simulink model "Meas_Noise_Test"  (R2022a)
settings: Solver=FixedStepAuto  StartTime=tspan(1)  StopTime=tspan(2)  FixedStep=Ts  RelTol=1e-9
undefined symbols (not defined in the file): Serial_Port, Standard_Devices, Ts
libraries: simulink_extras x4, sldrtlib x2, simulink x1, cstblocks x1
settings Model: SimulationMode=external  Creator=zachn  LastModifiedBy=domin
settings SolverCC: AlgebraicLoopSolver=TrustRegion
settings DataIOCC: SaveFormat=StructureWithTime  InspectSignalLogs=on
settings DebuggingCC: UnconnectedInputMsg=warning  UnconnectedOutputMsg=warning  UnconnectedLineMsg=warning  SFMachineParentedDataDiag=warning
settings HardwareCC: ProdBitPerLong=64  ProdHWDeviceType=Intel->x86-64 (Linux 64)
settings RTWCC: Description=Simulink Desktop Real-Time  SystemTargetFile=sldrt.tlc  TemplateMakefile=sldrt.tmf  RTWCompilerOptimization=on  DLArmComputeVersion=19.05
settings CodeAppCC: MaxIdLength=95
settings SimulinkDesktopRealTimeCC: TargetLibSuffix=_sldrt.a  TargetPreCompLibLocation=C:\Program Files\MATLAB\R2022a\toolbox\sldrt\lib\win64

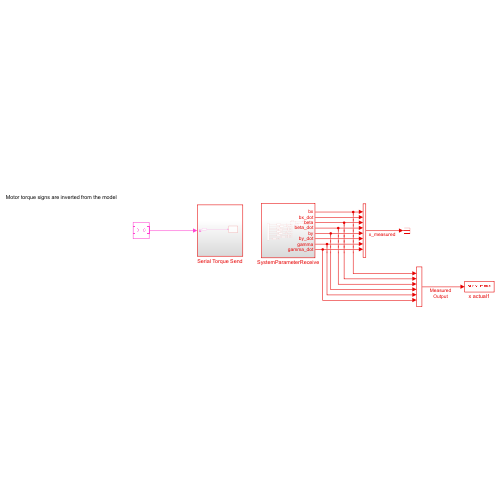
[thumbnail: Simulink's stored preview of the top-level diagram]
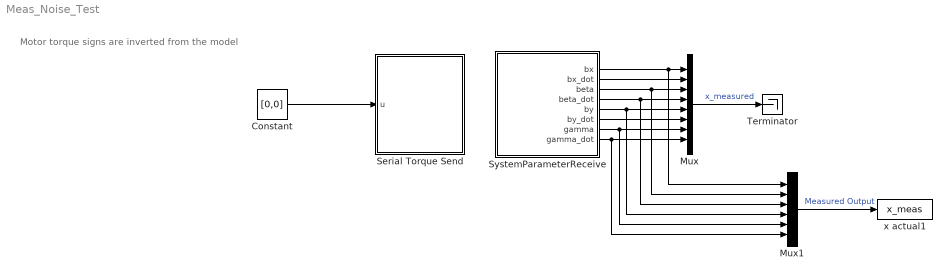
== system Meas_Noise_Test ==
  note: Motor torque signs are inverted from the model
  Constant : Constant  Value=[0,0]
  Mux : Mux  Inputs=8
  Mux1 : Mux  Inputs=6
  Serial Torque Send : Subsystem
  SystemParameterReceive : Subsystem
  Terminator : Terminator
  x actual1 : ToWorkspace  VariableName=x_meas  SampleTime=Ts
  wires:
  Constant/1 -> Serial Torque Send/1(u)
  SystemParameterReceive/6(by_dot) -> Mux/6
  SystemParameterReceive/2(bx_dot) -> Mux/2
  SystemParameterReceive/3(beta) -> Mux1/2, Mux/3
  SystemParameterReceive/5(by) -> Mux1/4, Mux/5
  Mux1/1 -> x actual1/1  "Measured Output"
  SystemParameterReceive/1(bx) -> Mux1/1, Mux/1
  SystemParameterReceive/8(gamma_dot) -> Mux1/6, Mux/8
  SystemParameterReceive/7(gamma) -> Mux1/5, Mux/7
  SystemParameterReceive/4(beta_dot) -> Mux1/3, Mux/4
  Mux/1 -> Terminator/1  "x_measured"

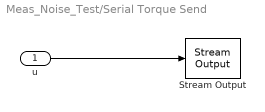
== system Meas_Noise_Test/Serial Torque Send ==
  u : Inport
  Stream Output : sldrtlib/Stream Output  SampleTime=Ts  MaxMissedTicks=10  ShowMissedTicks=off  YieldWhenWaiting=off  DrvName=Standard_Devices/Serial_Port  DrvAddress=6  DrvOptions=[115200 8 0 0 1 0 0 0]  PortSizes=2  FormatString='%g %g\n'  ShowReady=off  ShowError=off  InitialValue=[]  FinalValue=[]
      settings: AttributesFormatString=Serial Port [6]  SourceProductBaseCode=WT
  wires:
  u/1 -> Stream Output/1

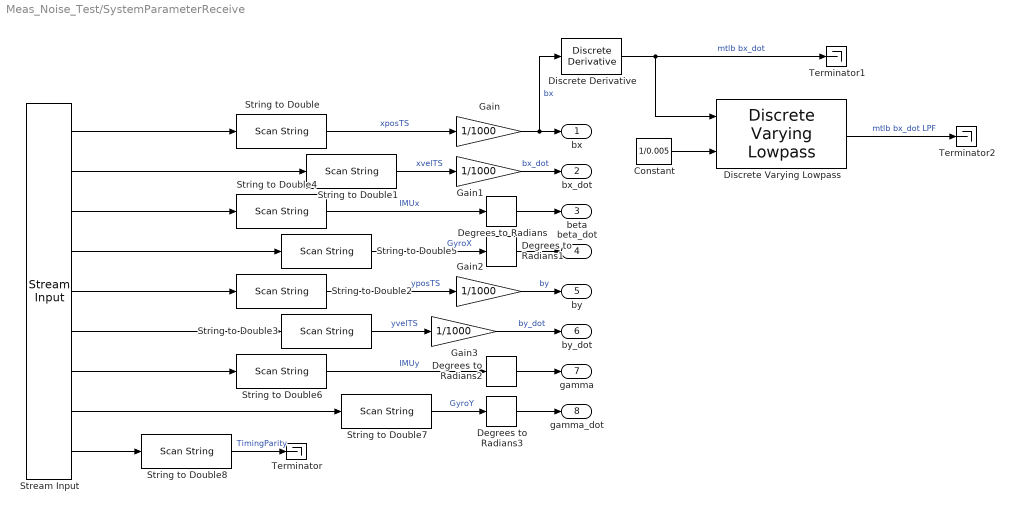
== system Meas_Noise_Test/SystemParameterReceive ==
  Constant : Constant  Value=1/0.005
  Degrees to Radians{,1..3} (4 alike) : simulink_extras/Transformations/Degrees to Radians
  Discrete Derivative : simulink/Discrete/Discrete Derivative  gainval=1.0  ICPrevScaledInput=0.0  OutMin=[]  OutMax=[]  OutDataType=fixdt(1, 16)  OutScaling=2^-10  DoSatur=off
  Discrete Varying Lowpass : cstblocks/Linear Parameter Varying/Discrete Varying Lowpass  N=4  w0=0  Ts=Ts
      settings: SourceProductBaseCode=CT
  Gain{,1..3} (4 alike) : Gain  Gain=1/1000  OutDataTypeStr=double
  Stream Input : sldrtlib/Stream Input  SampleTime=Ts  MaxMissedTicks=10  ShowMissedTicks=off  YieldWhenWaiting=on  DrvName=Standard_Devices/Serial_Port  DrvAddress=6  DrvOptions=[115200 8 0 0 1 0 0 0]  DataTypes={'string','string','string','string','string','string','string','string','string'}  FormatString='%s %s %s %s %s %s %s %s %s'  Terminator={'\r', '\n'}  ShowReady=off  ShowError=off
      settings: AttributesFormatString=Serial Port [6]  SourceProductBaseCode=WT
  String to Double : ScanString  Format="\"%d\""
  String to Double{1..8} (8 alike) : ScanString  Format="\"%lf\""
  Terminator : Terminator
  Terminator1 : Terminator
  Terminator2 : Terminator
  bx : Outport
  bx_dot : Outport  Port=2
  beta : Outport  Port=3
  beta_dot : Outport  Port=4
  by : Outport  Port=5
  by_dot : Outport  Port=6
  gamma : Outport  Port=7
  gamma_dot : Outport  Port=8
  wires:
  Stream Input/1 -> String to Double/1
  Stream Input/8 -> String to Double7/1
  Degrees to Radians3/1 -> gamma_dot/1
  Degrees to Radians2/1 -> gamma/1
  Stream Input/6 -> String to Double3/1
  Stream Input/9 -> String to Double8/1
  Stream Input/5 -> String to Double2/1
  String to Double8/1 -> Terminator/1  "TimingParity"
  Stream Input/7 -> String to Double6/1
  String to Double6/1 -> Degrees to Radians2/1  "IMUy"
  Stream Input/2 -> String to Double1/1
  String to Double1/1 -> Gain1/1  "xvelTS"
  Gain1/1 -> bx_dot/1  "bx_dot"
  Stream Input/4 -> String to Double5/1
  Stream Input/3 -> String to Double4/1
  Gain/1 -> Discrete Derivative/1, bx/1  "bx"
  String to Double/1 -> Gain/1  "xposTS"
  String to Double7/1 -> Degrees to Radians3/1  "GyroY"
  String to Double2/1 -> Gain2/1  "yposTS"
  Gain2/1 -> by/1  "by"
  Gain3/1 -> by_dot/1  "by_dot"
  String to Double3/1 -> Gain3/1  "yvelTS"
  Degrees to Radians1/1 -> beta_dot/1
  Degrees to Radians/1 -> beta/1
  String to Double4/1 -> Degrees to Radians/1  "IMUx"
  String to Double5/1 -> Degrees to Radians1/1  "GyroX"
  Discrete Derivative/1 -> Discrete Varying Lowpass/1, Terminator1/1  "mtlb bx_dot"
  Constant/1 -> Discrete Varying Lowpass/2
  Discrete Varying Lowpass/1 -> Terminator2/1  "mtlb bx_dot LPF"
